simulink model "BFSK_AWGN_BER"  (Simulink 6.5)
settings: Solver=VariableStepDiscrete  StartTime=0.0  StopTime=xSimulationTime  RelTol=1e-3
values from neighbouring files (symbols this model uses):
  BitRate = 10000    [Simulink_BFSK_RicianFading_BER.m]    (also in Simulink_Reileigh_BFSK_BER.m)
libraries: commdigbbndfm2 x2, commchan3 x1, commsink2 x1, commrandsrc2 x1
settings Model: Creator=Administrator  LastModifiedBy=Administrator

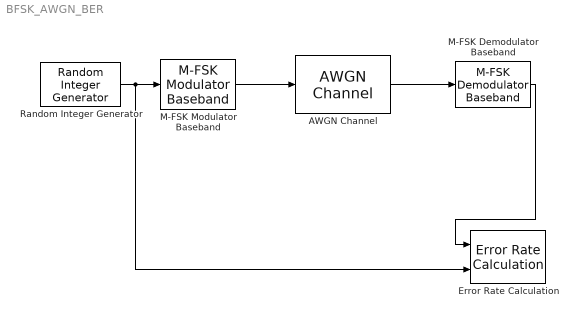
== system BFSK_AWGN_BER ==
  AWGN Channel : commchan3/AWGN Channel  SystemSampleTime=-1  seed=320  noiseMode="Signal to noise ratio  (SNR)"  EbNodB=10  EsNodB=10  SNRdB=SNR  bitsPerSym=1  Ps=1  Tsym=1  variance=1
  Error Rate Calculation : commsink2/Error Rate Calculation  N=0  st_delay=0  cp_mode=Entire frame  subframe=[]  PMode=Workspace  WsName=xErrorRate2  RsMode2=off  stop=off  numErr=100  maxBits=1e6
  M-FSK Demodulator Baseband : commdigbbndfm2/M-FSK Demodulator Baseband  M=2  OutType=Bit  Dec=Binary  freqSep=FrequencySeparation  numSamp=2  outDataType=double
  M-FSK Modulator Baseband : commdigbbndfm2/M-FSK Modulator Baseband  M=2  InType=Bit  Enc=Binary  freqSep=FrequencySeparation  phaseType=Continuous  numSamp=2  outDataType=double
  Random Integer Generator : commrandsrc2/Random Integer Generator  SystemSampleTime=-1  mul=2  seed=320  Ts=1/BitRate  frameBased=on  sampPerFrame=BitRate  orient=off  outDataType=double
  wires:
  Random Integer Generator/1 -> M-FSK Modulator Baseband/1, Error Rate Calculation/2
  AWGN Channel/1 -> M-FSK Demodulator Baseband/1
  M-FSK Modulator Baseband/1 -> AWGN Channel/1
  M-FSK Demodulator Baseband/1 -> Error Rate Calculation/1
